simulink model "coupled_model"  (R2014a)
settings: Solver=ode3  StartTime=0.0  StopTime=300  FixedStep=0.01  RelTol=1e-3
values from neighbouring files (symbols this model uses):
  G0 = Gb + p0    (= 276)    [Modified_Bergman.m]    (also in data.m = 287)
  Gb = 81    [Modified_Bergman.m]    (also in data.m = 92)
  I0 = Ib + 396    (= 411)    [Modified_Bergman.m]    (also in data.m = 300)
  Ib = 15    [Modified_Bergman.m]    (also in data.m = 7.3)
  p1 = 0.028735    [Modified_Bergman.m]    (also in data.m = 0.03082)
  p2 = 0.028344    [Modified_Bergman.m]    (also in data.m = 0.02093)
  p3 = 5.035E-5    (= 5.035e-05)    [Modified_Bergman.m]    (also in data.m = 1.06e-05)
  X0 = 0    [Modified_Bergman.m]    (also in data.m)
settings Model: Creator=sameer  LastModifiedBy=sameer

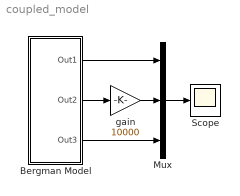
== system coupled_model ==
  "Bergman Model " : Subsystem
  Mux : Mux  Inputs=3
  "Scope " : Scope
      settings: SaveName=X3
  gain : Gain  Gain=10000
  wires:
  "Bergman Model "/1(Out1) -> Mux/1
  "Bergman Model "/2(Out2) -> gain/1
  "Bergman Model "/3(Out3) -> Mux/3
  Mux/1 -> "Scope "/1
  gain/1 -> Mux/2

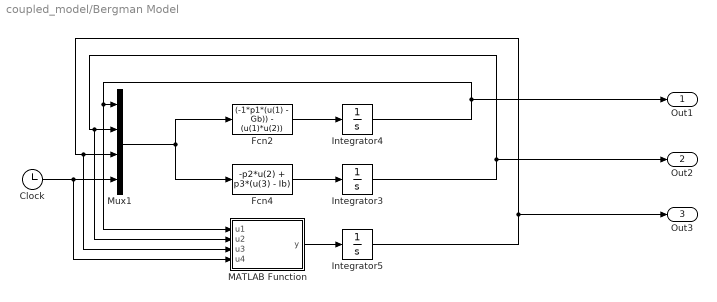
== system coupled_model/Bergman Model  ==
  Clock : Clock
  Fcn2 : Fcn  Expr=(-1*p1*(u(1) - Gb)) - (u(1)*u(2))
  Fcn4 : Fcn  Expr=-p2*u(2) + p3*(u(3) - Ib)
  Integrator3 : Integrator  InitialCondition=X0
  Integrator4 : Integrator  InitialCondition=G0
  Integrator5 : Integrator  InitialCondition=I0
  MATLAB Function : MATLAB Function  TreatAsAtomicUnit=on
  Mux1 : Mux
  Out1 : Outport
  Out2 : Outport  Port=2
  Out3 : Outport  Port=3
  wires:
  Clock/1 -> MATLAB Function/4(u4), Mux1/4
  MATLAB Function/1(y) -> Integrator5/1
  Integrator3/1 -> Out2/1, MATLAB Function/2(u2), Mux1/2
  Integrator4/1 -> Out1/1, MATLAB Function/1(u1), Mux1/1
  Fcn4/1 -> Integrator3/1
  Fcn2/1 -> Integrator4/1
  Mux1/1 -> Fcn4/1, Fcn2/1
  Integrator5/1 -> Out3/1, MATLAB Function/3(u3), Mux1/3

== matlab function coupled_model/Bergman Model /MATLAB Function ==
  data: u1 input; y output; u2 input; u3 input; u4 input
function y  = fcn(u1,u2,u3,u4)
p4 = 0.3;
p5 = 94;
p6 = 0.003349;
Ib = 7.3;

if(u1 - p5) > 0
    y = p6*(u1 - p5)*u4 - p4*(u3 - Ib);
else
    y = -p4*(u3 - Ib);
end
